simulink model "F550_FaultInjection"  (R2023b)
settings: Solver=FixedStepDiscrete  StartTime=0.0  StopTime=inf  FixedStep=1/100  RelTol=1e-3  EnableMultiTasking=on
undefined symbols (not defined in the file or in its folder): control, IDLEPWM, MC_PITCH_P, MC_PITCHRATE_D, MC_PITCHRATE_I, MC_PITCHRATE_P, MC_ROLL_P, MC_ROLLRATE_D, MC_ROLLRATE_I, MC_ROLLRATE_P, MC_YAW_P, MC_YAWRATE_D, MC_YAWRATE_I, MC_YAWRATE_P, MPC_XY_P, MPC_XY_VEL_MAX, MPC_Z_D, MPC_Z_I, MPC_Z_P, MPC_Z_VEL_D_ACC, MPC_Z_VEL_I_ACC, MPC_Z_VEL_MAX_DN, MPC_Z_VEL_MAX_UP, MPC_Z_VEL_P_ACC, noutputs, output, pitch, pitch_body, roll, roll_body, SampleTime, TargetHardware, thrust_body, timestamp, x, y, yaw, yaw_body, z
libraries: px4lib x45, px4uORBlib x19, slpidlib x10, simulink x9, px4Utilslib x5, simulink_extras x5, px4Sensorslib x3, uavalgslib x3, sharedutil x1, sharedtransform x1
(part 1 of 4)
settings Model: ExtModeTrigDuration=10  Creator=The MathWorks, Inc.  LastModifiedBy=UASG
settings SolverCC: PositivePriorityOrder=on  MaxZcPerStep=1
settings OptimizationCC: StrengthReduction=on  PassReuseOutputArgsAs=Individual arguments  ZeroExternalMemoryAtStartup=off  ZeroInternalMemoryAtStartup=off  MaxStackSize=64  OptimizeBlockOrder=speed  OptimizationPriority=Speed  OptimizationCustomize=off  MultiThreadedLoops=on  EfficientTunableParamExpr=on
settings DebuggingCC: ParameterTunabilityLossMsg=error
settings HardwareCC: ProdBitPerPointer=32  ProdBitPerSizeT=32  ProdBitPerPtrDiffT=32  ProdLargestAtomicInteger=Long  ProdLargestAtomicFloat=Double  ProdWordSize=32  ProdLongLongMode=on  ProdHWDeviceType=ARM Compatible->ARM Cortex
settings ModelReferenceCC: EnableRefExpFcnMdlSchedulingChecks=on
settings SFSimCC: MATLABDynamicMemAlloc=off  SimTargetLang=C++
settings RTWCC: Description=Embedded Coder  SystemTargetFile=ert.tlc  HardwareBoard=PX4 Cube Orange  TLCOptions="-aInlineSetEventsForThisBaseRateFcn=TLC_FALSE -aSuppressMultiTaskScheduler=TLC_FALSE  -aRateBasedStepFcn=0"  TemplateMakefile=ert_default_tmf  GenerateReport=on  Toolchain=GNU Tools for PX4 Autopilots  BuildConfiguration=Faster Runs  LaunchReport=on  TargetLang=C++  DLArmComputeVersion=19.05
settings CodeAppCC: ForceParamTrailComments=on  IgnoreCustomStorageClasses=off  MaxIdLength=63  OperatorAnnotations=on  SimulinkDataObjDesc=on  SFDataObjDesc=on  InsertBlockDesc=on
settings ERTTargetCC: ExtModeTransport=3  ExtModeStaticAlloc=on  ExtModeStaticAllocSize=1024  ExtModeMexFile=ext_xcp  ExtModeIntrfLevel=Level2 - Open

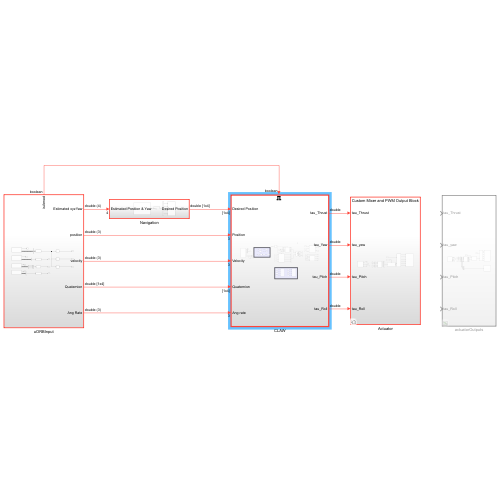
[thumbnail: Simulink's stored preview of the top-level diagram]
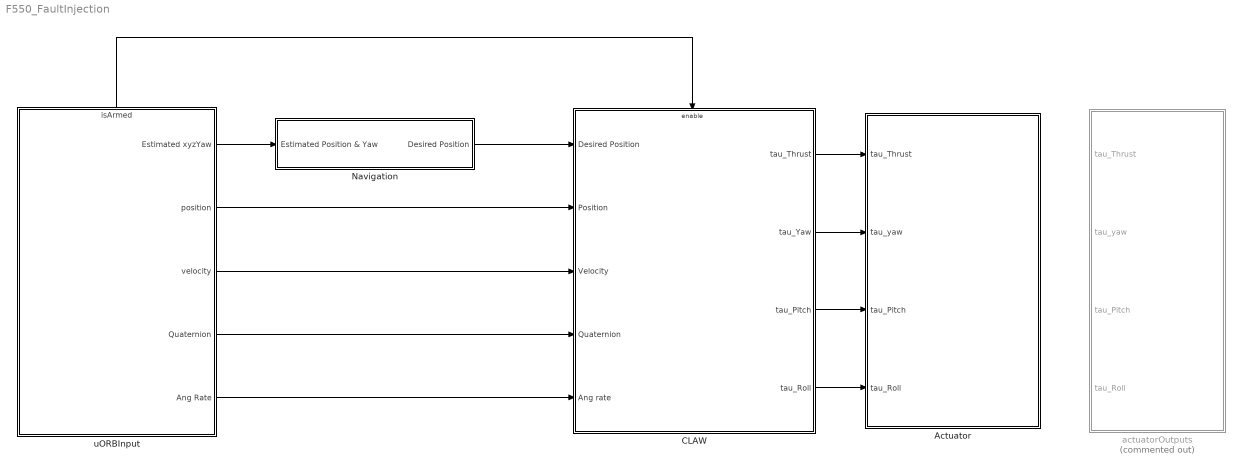
== system F550_FaultInjection ==
  Actuator : Subsystem  Variant=on
  CLAW : Subsystem  RTWFcnName=CLAW
      settings: RTWSystemCode=Nonreusable function  RTWFcnNameOpts=Use subsystem name  RTWFileNameOpts=Use subsystem name
  Navigation : Subsystem
      settings: RTWSystemCode=Nonreusable function  RTWFcnNameOpts=Use subsystem name  RTWFileNameOpts=Use subsystem name
  actuatorOutputs : Subsystem  Commented=on  TreatAsAtomicUnit=on
      settings: RTWSystemCode=Nonreusable function  RTWFcnNameOpts=Use subsystem name  RTWFileNameOpts=Use subsystem name
  uORBInput : Subsystem
      settings: RTWSystemCode=Nonreusable function  RTWFcnNameOpts=Use subsystem name  RTWFileNameOpts=Use subsystem name  PortSchema="{\"entries\":[{\"content\":{\"sides\":[{\"content\":{},\"type\":\"ConnectorPlacement.EquallySpacedRectSide\",\"uuid\":\"c9847de1-a0fb-4f12-b9ba-7a711e150495\"},{\"content\":{\"connectorIds\":[\"Out1\",\"Out2\",\"Out3\",\"Out4\",\"Out5\"],\"side\":\"RIGHT\"},\"type\":\"ConnectorPlacement.EquallySpacedRectSide\",\"uuid\":\"c0766eaa-9e51-4014-aa9e-b3d4f69fc081\"},{\"content\":{\"connectorIds\":[\"Out6\"],\"side\":\"TOP\"},\"type\":\"ConnectorPlacement.EquallySpacedRectSide\",\"uuid\":\"9ded9b51-a7f6-4f6f-b66b-95ea3c1db3ad\"}]},\"type\":\"ConnectorPlacement.EquallySpacedConnector\",\"uuid\":\"83553f6c-d7c4-4220-9d3b-5711d4bd470c\"}],\"packageUris\":[\"http://schema.mathworks.com/mf0/Connector/R2020b\"],\"version\":\"1.0\"}"
  wires:
  uORBInput/1(Estimated xyzYaw) -> Navigation/1(Estimated Position & Yaw)
  CLAW/4(tau_Roll) -> Actuator/4(tau_Roll)
  CLAW/3(tau_Pitch) -> Actuator/3(tau_Pitch)
  CLAW/2(tau_Yaw) -> Actuator/2(tau_yaw)
  CLAW/1(tau_Thrust) -> Actuator/1(tau_Thrust)
  Navigation/1(Desired Position) -> CLAW/1(Desired Position)
  uORBInput/2(position) -> CLAW/2(Position)
  uORBInput/3(velocity) -> CLAW/3(Velocity)
  uORBInput/4(Quaternion) -> CLAW/4(Quaternion)
  uORBInput/5(Ang Rate) -> CLAW/5(Ang rate)
  uORBInput/6(isArmed) -> CLAW/Enable

== system F550_FaultInjection/Actuator ==
  tau_Thrust : Inport
  tau_yaw : Inport  Port=2
  tau_Pitch : Inport  Port=3
  tau_Roll : Inport  Port=4
  Custom Mixer and PWM Output Block : Subsystem  VariantControl=useCustomMixer == true
  PX4 Mixer and actuator_controls_0 topic : Subsystem  VariantControl=useCustomMixer == false

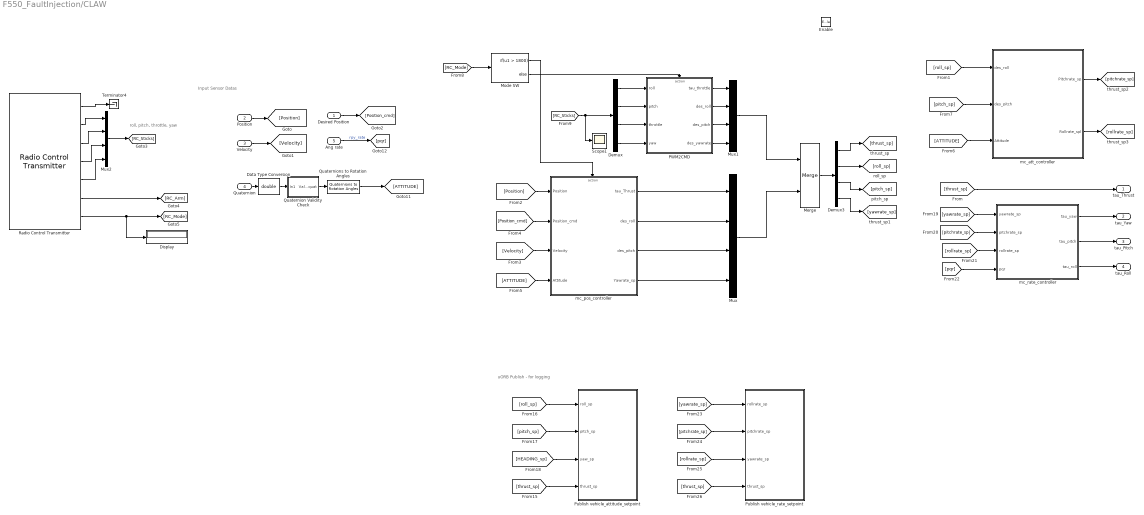
== system F550_FaultInjection/CLAW ==
  note: roll, pitch, throttle, yaw
  note: Input Sensor Datas
  note: uORB Publish - for logging
  Desired Position : Inport
  Position : Inport  Port=2
  Velocity : Inport  Port=3
  Quaternion : Inport  Port=4
  Ang rate : Inport  Port=5
  Enable : EnablePort
  Data Type Conversion : DataTypeConversion  OutDataTypeStr=double  SaturateOnIntegerOverflow=off  RndMeth=Floor
  Demux : Demux
  Demux3 : Demux
  Display : Display
  Merge : Merge
  Mode SW : If  IfExpression=u1 > 1800
  Mux : Mux
  Mux1 : Mux
  Mux2 : Mux
  PWM2CMD : Subsystem
  Publish vehicle_attitude_setpoint : Subsystem
  Publish vehicle_rate_setpoint : Subsystem
  Quaternion Validity Check : Subsystem
  Quaternions to Rotation Angles : sharedtransform/Quaternions to Rotation Angles  rotationOrder=ZYX  aMode=aMode
  Radio Control Transmitter : px4Sensorslib/Radio Control Transmitter  channel1=on  channel2=on  channel3=on  channel4=on  channel5=on  channel6=on  channel7=off  channel8=off  channel_count=off  rssi=off  rc_input_source=off  timestamp_last_signal=off  time_stamp=off  sampleTime=-1  BlockingMode=off  BlockTimeout=5
  Scope1 : Scope
  Terminator4 : Terminator
  mc_att_controller : Subsystem
      settings: RTWSystemCode=Nonreusable function  RTWFcnNameOpts=Use subsystem name  RTWFileNameOpts=Use subsystem name
  mc_pos_controller : Subsystem
      settings: RTWSystemCode=Nonreusable function  RTWFcnNameOpts=Use subsystem name  RTWFileNameOpts=Use subsystem name
  mc_rate_controller : Subsystem
      settings: RTWSystemCode=Nonreusable function  RTWFcnNameOpts=Use subsystem name  RTWFileNameOpts=Use subsystem name
  tau_Thrust : Outport
  tau_Yaw : Outport  Port=2
  tau_Pitch : Outport  Port=3
  tau_Roll : Outport  Port=4
  wires:
  [rollrate_sp] -> Publish vehicle_rate_setpoint/3(yawrate_sp)
  [thrust_sp] -> Publish vehicle_rate_setpoint/4(thrust_sp)
  [yawrate_sp] -> Publish vehicle_rate_setpoint/1(rollrate_sp)
  [yawrate_sp] -> mc_rate_controller/1(yawrate_sp)
  Position/1 -> [Position]
  [pqr] -> mc_rate_controller/4(pqr)
  mc_rate_controller/3(tau_roll) -> tau_Roll/1
  [pitchrate_sp] -> mc_rate_controller/2(pitchrate_sp)
  mc_rate_controller/1(tau_yaw) -> tau_Yaw/1
  mc_att_controller/1(Pitchrate_sp) -> [pitchrate_sp]
  [thrust_sp] -> Publish vehicle_attitude_setpoint/4(thrust_sp)
  [pitchrate_sp] -> Publish vehicle_rate_setpoint/2(pitchrate_sp)
  Quaternion/1 -> Data Type Conversion/1
  mc_rate_controller/2(tau_pitch) -> tau_Pitch/1
  Desired Position/1 -> [Position_cmd]
  Ang rate/1 -> [pqr]  "rpy_rate"
  [thrust_sp] -> tau_Thrust/1
  [rollrate_sp] -> mc_rate_controller/3(rollrate_sp)
  Velocity/1 -> [Velocity]
  mc_att_controller/2(Rollrate_spl) -> [rollrate_sp]
  Quaternion Validity Check/1(Valid quat) -> Quaternions to Rotation Angles/1
  [pitch_sp] -> Publish vehicle_attitude_setpoint/2(pitch_sp)
  [HEADING_sp] -> Publish vehicle_attitude_setpoint/3(yaw_sp)
  [roll_sp] -> Publish vehicle_attitude_setpoint/1(roll_sp)
  Data Type Conversion/1 -> Quaternion Validity Check/1(In1)
  Merge/1 -> Demux3/1
  Demux3/1 -> [thrust_sp]
  Demux3/2 -> [roll_sp]
  Demux3/3 -> [pitch_sp]
  Demux3/4 -> [yawrate_sp]
  [Position] -> mc_pos_controller/1(Position)
  [Velocity] -> mc_pos_controller/3(Velocity)
  [Position_cmd] -> mc_pos_controller/2(Position_cmd)
  [ATTITUDE] -> mc_pos_controller/4(Attitude)
  mc_pos_controller/1(tau_Thrust) -> Mux/1
  mc_pos_controller/2(des_roll) -> Mux/2
  mc_pos_controller/3(des_pitch) -> Mux/3
  mc_pos_controller/4(Yawrate_sp) -> Mux/4
  Mux/1 -> Merge/2
  Mux1/1 -> Merge/1
  [roll_sp] -> mc_att_controller/1(des_roll)
  [ATTITUDE] -> mc_att_controller/3(Attitude)
  [pitch_sp] -> mc_att_controller/2(des_pitch)
  PWM2CMD/1(tau_throttle) -> Mux1/1
  PWM2CMD/2(des_roll) -> Mux1/2
  PWM2CMD/3(des_pitch) -> Mux1/3
  PWM2CMD/4(des_yawrate) -> Mux1/4
  Quaternions to Rotation Angles/1 -> [ATTITUDE]
  [RC_Mode] -> Mode SW/1
  Radio Control Transmitter/6 -> [RC_Arm]
  Radio Control Transmitter/1 -> Terminator4/1
  Radio Control Transmitter/7 -> Display/1, [RC_Mode]
  Radio Control Transmitter/2 -> Mux2/1
  Radio Control Transmitter/3 -> Mux2/2
  Radio Control Transmitter/4 -> Mux2/3
  Radio Control Transmitter/5 -> Mux2/4
  Mux2/1 -> [RC_Sticks]
  Demux/1 -> PWM2CMD/1(roll)
  Demux/2 -> PWM2CMD/2(pitch)
  Demux/3 -> PWM2CMD/3(throttle)
  Demux/4 -> PWM2CMD/4(yaw)
  [RC_Sticks] -> Scope1/1, Demux/1
  Mode SW/2 -> PWM2CMD/Action
  Mode SW/1 -> mc_pos_controller/Action

== system F550_FaultInjection/Navigation ==
  Estimated Position & Yaw : Inport
  Demux : Demux
  Quadcopter Navigation Algorithm : Subsystem  Variant=on
  uORB Publish : Subsystem
  Desired Position : Outport
  wires:
  Quadcopter Navigation Algorithm/1(Desired Position) -> Demux/1, Desired Position/1
  Estimated Position & Yaw/1 -> Quadcopter Navigation Algorithm/1(Current Position)
  Demux/1 -> uORB Publish/1(x_sp)
  Demux/2 -> uORB Publish/2(y_sp)
  Demux/3 -> uORB Publish/3(z_sp)
  Demux/4 -> uORB Publish/4(heading_sp)

== system F550_FaultInjection/actuatorOutputs ==
  tau_Thrust : Inport
  tau_yaw : Inport  Port=2
  tau_Pitch : Inport  Port=3
  tau_Roll : Inport  Port=4
  Emergency Kill : Subsystem
  Fault Injection Module : Subsystem  Variant=on
  Gain : Gain  Gain=5
  Gain1 : Gain  Gain=5
  Gain2 : Gain  Gain=10
  MATLAB Function : MATLAB Function  TreatAsAtomicUnit=on
  Mux : Mux  Inputs=6
  Mux1 : Mux
  Radio Control Transmitter : px4Sensorslib/Radio Control Transmitter  channel1=off  channel2=off  channel3=off  channel4=off  channel5=off  channel6=on  channel7=on  channel8=off  channel_count=off  rssi=off  rc_input_source=off  timestamp_last_signal=off  time_stamp=off  sampleTime=-1  BlockingMode=off  BlockTimeout=5
  Saturation : Saturate  UpperLimit=1  LowerLimit=0
  Saturation1 : Saturate  UpperLimit=1  LowerLimit=-1
  Saturation2 : Saturate  UpperLimit=1  LowerLimit=-1
  Saturation3 : Saturate  UpperLimit=1  LowerLimit=-1
  Terminator : Terminator
  uORB_actuator_controls : Subsystem
  uORB_actuator_outputs : Subsystem
  wires:
  MATLAB Function/1(M1) -> Mux/1
  Radio Control Transmitter/1 -> Terminator/1
  MATLAB Function/2(M2) -> Mux/2
  tau_Thrust/1 -> Saturation/1  "thrust cmd"
  tau_Pitch/1 -> Gain1/1  "pitch cmd"
  MATLAB Function/3(M3) -> Mux/3
  [Kill] -> Emergency Kill/1(Kill)
  MATLAB Function/6(M6) -> Mux/6
  tau_yaw/1 -> Gain2/1
  Radio Control Transmitter/2 -> [InjectFault]
  Radio Control Transmitter/3 -> [Kill]
  tau_Roll/1 -> Gain/1  "roll_cmd"
  MATLAB Function/4(M4) -> Mux/4
  MATLAB Function/5(M5) -> Mux/5
  [InjectFault] -> Fault Injection Module/1(Inject Fault)
  Mux/1 -> Fault Injection Module/2(PWM_IN)
  Fault Injection Module/1(PWM_OUT) -> Emergency Kill/2(PWM_IN)
  Mux1/1 -> uORB_actuator_controls/1(actuator_control_out)
  Saturation/1 -> Mux1/4, MATLAB Function/4(Thrust)
  Saturation1/1 -> Mux1/3, MATLAB Function/3(Yaw)
  Saturation2/1 -> Mux1/2, MATLAB Function/2(Pitch)
  Saturation3/1 -> Mux1/1, MATLAB Function/1(Roll)
  Gain/1 -> Saturation3/1
  Gain1/1 -> Saturation2/1
  Gain2/1 -> Saturation1/1
  Emergency Kill/1(M1_OUT) -> uORB_actuator_outputs/1(Ch1)
  Emergency Kill/2(M2_OUT) -> uORB_actuator_outputs/2(Ch2)
  Emergency Kill/3(M3_OUT) -> uORB_actuator_outputs/3(Ch3)
  Emergency Kill/4(M4_OUT) -> uORB_actuator_outputs/4(Ch4)
  Emergency Kill/5(M5_OUT) -> uORB_actuator_outputs/5(Ch5)
  Emergency Kill/6(M6_OUT) -> uORB_actuator_outputs/6(Ch6)

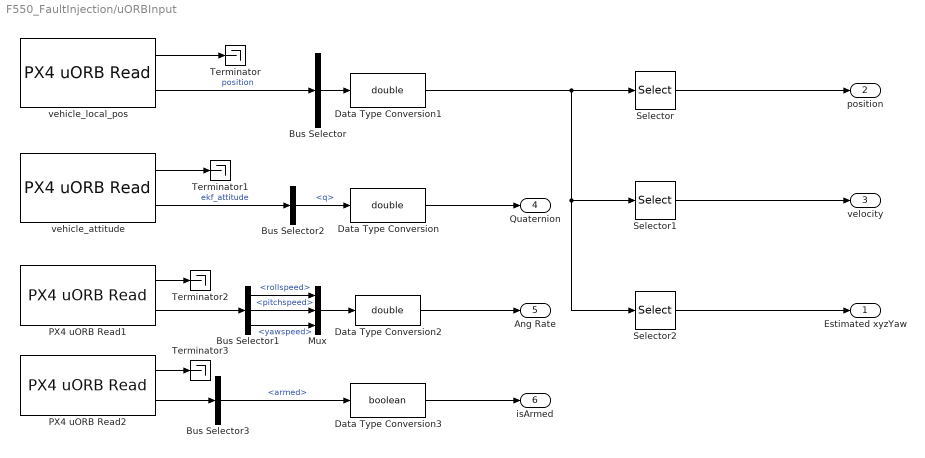
== system F550_FaultInjection/uORBInput ==
  Bus Selector : BusSelector  OutputSignals=x,y,z,vx,vy,vz,heading  OutputAsBus=on
  Bus Selector1 : BusSelector  OutputSignals=rollspeed,pitchspeed,yawspeed
  Bus Selector2 : BusSelector  OutputSignals=q
  Bus Selector3 : BusSelector  OutputSignals=armed
  Data Type Conversion : DataTypeConversion  OutDataTypeStr=double  SaturateOnIntegerOverflow=off  RndMeth=Floor
  Data Type Conversion1 : DataTypeConversion  OutDataTypeStr=double  SaturateOnIntegerOverflow=off  RndMeth=Floor
  Data Type Conversion2 : DataTypeConversion  OutDataTypeStr=double  SaturateOnIntegerOverflow=off  RndMeth=Floor
  Data Type Conversion3 : DataTypeConversion  OutDataTypeStr=boolean  SaturateOnIntegerOverflow=off  RndMeth=Floor
  Mux : Mux  Inputs=3
  PX4 uORB Read1 : px4uORBlib/PX4 uORB Read  uORBTopic=vehicle_odometry  selectInstance=vehicle_odometry  SampleTime=-1  BlockingMode=off  BlockTimeout=1e-3
  PX4 uORB Read2 : px4uORBlib/PX4 uORB Read  uORBTopic=actuator_armed  selectInstance=actuator_armed  SampleTime=-1  BlockingMode=off  BlockTimeout=1e-3
  Selector : Selector  InputPortWidth=7  IndexOptions=Index vector (dialog)  Indices=[1:3]  OutputSizes=1
  Selector1 : Selector  InputPortWidth=7  IndexOptions=Index vector (dialog)  Indices=[4:6]  OutputSizes=1
  Selector2 : Selector  InputPortWidth=7  IndexOptions=Index vector (dialog)  Indices=[1 2 3 7]  OutputSizes=1
  Terminator{,1..3} (4 alike) : Terminator
  vehicle_attitude : px4uORBlib/PX4 uORB Read  uORBTopic=vehicle_attitude  selectInstance=vehicle_attitude  SampleTime=-1  BlockingMode=off  BlockTimeout=1e-3
  vehicle_local_pos : px4uORBlib/PX4 uORB Read  uORBTopic=vehicle_local_position  selectInstance=vehicle_local_position  SampleTime=-1  BlockingMode=off  BlockTimeout=1e-3
  Estimated xyzYaw : Outport
  position : Outport  Port=2
  velocity : Outport  Port=3
  Quaternion : Outport  Port=4
  Ang Rate : Outport  Port=5
  isArmed : Outport  Port=6
  wires:
  Bus Selector2/1 -> Data Type Conversion/1  "<q>"
  vehicle_local_pos/2 -> Bus Selector/1  "position"
  Data Type Conversion1/1 -> Selector1/1, Selector2/1, Selector/1
  vehicle_attitude/1 -> Terminator1/1
  vehicle_attitude/2 -> Bus Selector2/1  "ekf_attitude"
  vehicle_local_pos/1 -> Terminator/1
  Bus Selector/1 -> Data Type Conversion1/1
  PX4 uORB Read1/1 -> Terminator2/1
  PX4 uORB Read1/2 -> Bus Selector1/1
  Mux/1 -> Data Type Conversion2/1
  PX4 uORB Read2/1 -> Terminator3/1
  Bus Selector3/1 -> Data Type Conversion3/1  "<armed>"
  PX4 uORB Read2/2 -> Bus Selector3/1
  Bus Selector1/1 -> Mux/1  "<rollspeed>"
  Bus Selector1/2 -> Mux/2  "<pitchspeed>"
  Bus Selector1/3 -> Mux/3  "<yawspeed>"
  Selector/1 -> position/1
  Selector1/1 -> velocity/1
  Selector2/1 -> Estimated xyzYaw/1
  Data Type Conversion/1 -> Quaternion/1
  Data Type Conversion2/1 -> Ang Rate/1
  Data Type Conversion3/1 -> isArmed/1

== system F550_FaultInjection/Actuator/Custom Mixer and PWM Output Block ==
  tau_Thrust : Inport
  tau_yaw : Inport  Port=2
  tau_Pitch : Inport  Port=3
  tau_Roll : Inport  Port=4
  Emergency Kill : Subsystem
  Fault_Injection : Subsystem
      settings: PortSchema="{\"entries\":[{\"content\":{\"sides\":[{\"content\":{\"connectorIds\":[\"In1\"]},\"type\":\"ConnectorPlacement.EquallySpacedRectSide\",\"uuid\":\"fab26c65-8d77-46b7-b375-2033d08e8306\"},{\"content\":{\"connectorIds\":[\"Out1\"],\"side\":\"RIGHT\"},\"type\":\"ConnectorPlacement.EquallySpacedRectSide\",\"uuid\":\"bc3f50bd-e170-4b75-8089-4f92da68e83e\"},{\"content\":{\"connectorIds\":[\"In2\"],\"side\":\"TOP\"},\"type\":\"ConnectorPlacement.EquallySpacedRectSide\",\"uuid\":\"873ada90-6f93-48ab-a701-a52d28357753\"}]},\"type\":\"ConnectorPlacement.EquallySpacedConnector\",\"uuid\":\"201be8b3-bff4-4924-8e0c-28e5fee33d1c\"}],\"packageUris\":[\"http://schema.mathworks.com/mf0/Connector/R2020b\"],\"version\":\"1.0\"}"
  Gain : Gain  Gain=5
  Gain1 : Gain  Gain=5
  Gain2 : Gain  Gain=10
  Gain3 : Gain
  MATLAB Function : MATLAB Function  TreatAsAtomicUnit=on
  Mux : Mux  Inputs=6
  Radio Control Transmitter : px4Sensorslib/Radio Control Transmitter  channel1=off  channel2=off  channel3=off  channel4=off  channel5=off  channel6=off  channel7=on  channel8=on  channel_count=off  rssi=off  rc_input_source=off  timestamp_last_signal=off  time_stamp=off  sampleTime=-1  BlockingMode=off  BlockTimeout=5
  Subsystem : Subsystem
  Terminator : Terminator
  wires:
  Radio Control Transmitter/2 -> [Kill]
  [InjectFault] -> Fault_Injection/2(Inject Fault)
  Fault_Injection/1(PWM_OUT) -> Emergency Kill/2(PWM_IN)
  [Kill] -> Emergency Kill/1(Kill)
  Radio Control Transmitter/3 -> [InjectFault]
  Radio Control Transmitter/1 -> Terminator/1
  Emergency Kill/2(M2_OUT) -> Subsystem/2(Ch2)
  Emergency Kill/3(M3_OUT) -> Subsystem/3(Ch3)
  Emergency Kill/4(M4_OUT) -> Subsystem/4(Ch4)
  Emergency Kill/5(M5_OUT) -> Subsystem/5(Ch5)
  Emergency Kill/6(M6_OUT) -> Subsystem/6(Ch6)
  Emergency Kill/1(M1_OUT) -> Subsystem/1(Ch1)
  tau_Thrust/1 -> Gain3/1  "thrust cmd"
  tau_Roll/1 -> Gain/1  "roll_cmd"
  tau_Pitch/1 -> Gain1/1  "pitch cmd"
  tau_yaw/1 -> Gain2/1
  MATLAB Function/1(M1) -> Mux/1
  MATLAB Function/2(M2) -> Mux/2
  MATLAB Function/3(M3) -> Mux/3
  MATLAB Function/4(M4) -> Mux/4
  MATLAB Function/5(M5) -> Mux/5
  MATLAB Function/6(M6) -> Mux/6
  Mux/1 -> Fault_Injection/1(PWM_IN)
  Gain/1 -> MATLAB Function/1(Roll)
  Gain1/1 -> MATLAB Function/2(Pitch)
  Gain2/1 -> MATLAB Function/3(Yaw)
  Gain3/1 -> MATLAB Function/4(Thrust)

== system F550_FaultInjection/Actuator/PX4 Mixer and actuator_controls_0 topic ==
  tau_Thrust : Inport
  tau_yaw : Inport  Port=2
  tau_Pitch : Inport  Port=3
  tau_Roll : Inport  Port=4
  Armed : Inport  Port=5
  Bus Assignment : BusAssignment  AssignedSignals=control
  Constant : Constant  Value=zeros(4,1)
  Data Type Conversion : DataTypeConversion  SaturateOnIntegerOverflow=off  RndMeth=Floor
  Mux : Mux  Inputs=5
  PX4 uORB Message : px4uORBlib/PX4 uORB Message  uORBTopic=actuator_controls  SampleTime=inf  selectInstance=vehicle_gps_position
  PX4 uORB Write : px4uORBlib/PX4 uORB Write  uORBTopic=actuator_controls  selectInstance=actuator_controls_0  MessageQueueLen=1
  Terminator : Terminator
  wires:
  Bus Assignment/1 -> PX4 uORB Write/1
  tau_yaw/1 -> Mux/3
  Data Type Conversion/1 -> Bus Assignment/2
  tau_Roll/1 -> Mux/1  "roll_cmd"
  PX4 uORB Message/1 -> Bus Assignment/1
  Mux/1 -> Data Type Conversion/1
  Constant/1 -> Mux/5
  tau_Pitch/1 -> Mux/2  "pitch cmd"
  tau_Thrust/1 -> Mux/4  "thrust cmd"
  Armed/1 -> Terminator/1

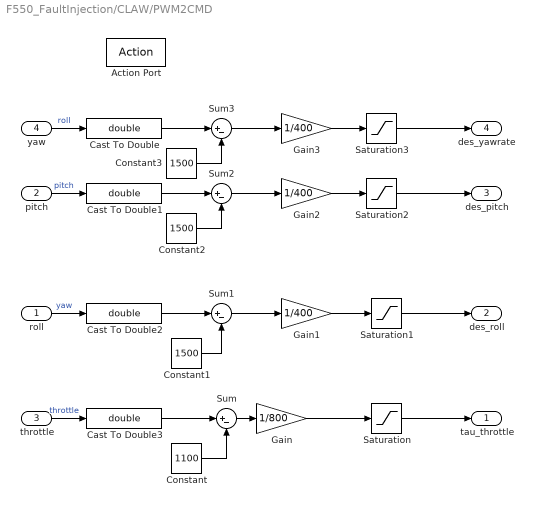
== system F550_FaultInjection/CLAW/PWM2CMD ==
  roll : Inport
  pitch : Inport  Port=2
  throttle : Inport  Port=3
  yaw : Inport  Port=4
  Action Port : ActionPort  ActionPortLabel=else
  Cast To Double{,1..3} (4 alike) : DataTypeConversion  OutDataTypeStr=double  SaturateOnIntegerOverflow=off  RndMeth=Floor
  Constant : Constant  Value=1100
  Constant1 : Constant  Value=1500
  Constant2 : Constant  Value=1500
  Constant3 : Constant  Value=1500
  Gain : Gain  Gain=1/800
  Gain1 : Gain  Gain=1/400
  Gain2 : Gain  Gain=1/400
  Gain3 : Gain  Gain=1/400
  Saturation : Saturate  UpperLimit=1  LowerLimit=0
  Saturation1 : Saturate  UpperLimit=1  LowerLimit=-1
  Saturation2 : Saturate  UpperLimit=1  LowerLimit=-1
  Saturation3 : Saturate  UpperLimit=1  LowerLimit=-1
  Sum{,1..3} (4 alike) : Sum  Inputs=|+-
  tau_throttle : Outport
  des_roll : Outport  Port=2
  des_pitch : Outport  Port=3
  des_yawrate : Outport  Port=4
  wires:
  Gain/1 -> Saturation/1
  Constant1/1 -> Sum1/2
  throttle/1 -> Cast To Double3/1  "throttle"
  yaw/1 -> Cast To Double/1  "roll"
  Constant3/1 -> Sum3/2
  Gain2/1 -> Saturation2/1
  pitch/1 -> Cast To Double1/1  "pitch"
  Constant2/1 -> Sum2/2
  roll/1 -> Cast To Double2/1  "yaw"
  Sum1/1 -> Gain1/1
  Sum2/1 -> Gain2/1
  Gain3/1 -> Saturation3/1
  Constant/1 -> Sum/2
  Sum/1 -> Gain/1
  Sum3/1 -> Gain3/1
  Gain1/1 -> Saturation1/1
  Saturation3/1 -> des_yawrate/1
  Saturation2/1 -> des_pitch/1
  Saturation1/1 -> des_roll/1
  Saturation/1 -> tau_throttle/1
  Cast To Double/1 -> Sum3/1
  Cast To Double1/1 -> Sum2/1
  Cast To Double2/1 -> Sum1/1
  Cast To Double3/1 -> Sum/1

== system F550_FaultInjection/CLAW/Publish vehicle_attitude_setpoint ==
  note: bX : Body frame ,X axis
  roll_sp : Inport
  pitch_sp : Inport  Port=2
  yaw_sp : Inport  Port=3
  thrust_sp : Inport  Port=4
  Bus Assignment : BusAssignment  AssignedSignals=timestamp,roll_body,pitch_body,yaw_body,thrust_body
  Data Type Conversion{,1..3} (4 alike) : DataTypeConversion  OutDataTypeStr=single  SaturateOnIntegerOverflow=off  RndMeth=Floor
  Mux : Mux  Inputs=3
  PX4 Timestamp : px4Utilslib/PX4 Timestamp  SampleTime=-1
  PX4 uORB Message : px4uORBlib/PX4 uORB Message  uORBTopic=vehicle_attitude_setpoint  SampleTime=-1  selectInstance=actuator_controls
  PX4 uORB Write : px4uORBlib/PX4 uORB Write  uORBTopic=vehicle_attitude_setpoint  selectInstance=vehicle_attitude_setpoint  MessageQueueLen=1
  thrust_sp_bX : Constant  Value=0
  thrust_sp_bY : Constant  Value=0
  wires:
  PX4 Timestamp/1 -> Bus Assignment/2
  Bus Assignment/1 -> PX4 uORB Write/1
  PX4 uORB Message/1 -> Bus Assignment/1
  roll_sp/1 -> Data Type Conversion/1
  pitch_sp/1 -> Data Type Conversion1/1
  yaw_sp/1 -> Data Type Conversion2/1
  Data Type Conversion/1 -> Bus Assignment/3
  Data Type Conversion1/1 -> Bus Assignment/4
  Data Type Conversion2/1 -> Bus Assignment/5
  thrust_sp_bX/1 -> Mux/1
  thrust_sp_bY/1 -> Mux/2
  thrust_sp/1 -> Mux/3
  Mux/1 -> Data Type Conversion3/1
  Data Type Conversion3/1 -> Bus Assignment/6

== system F550_FaultInjection/CLAW/Publish vehicle_rate_setpoint ==
  note: bX : Body frame ,X axis
  rollrate_sp : Inport
  pitchrate_sp : Inport  Port=2
  yawrate_sp : Inport  Port=3
  thrust_sp : Inport  Port=4
  Bus Assignment : BusAssignment  AssignedSignals=timestamp,roll,pitch,yaw,thrust_body
  Data Type Conversion{,1..3} (4 alike) : DataTypeConversion  OutDataTypeStr=single  SaturateOnIntegerOverflow=off  RndMeth=Floor
  Mux : Mux  Inputs=3
  PX4 Timestamp : px4Utilslib/PX4 Timestamp  SampleTime=-1
  PX4 uORB Message : px4uORBlib/PX4 uORB Message  uORBTopic=vehicle_rates_setpoint  SampleTime=-1  selectInstance=vehicle_rates_setpoint
  PX4 uORB Write : px4uORBlib/PX4 uORB Write  uORBTopic=vehicle_rates_setpoint  selectInstance=vehicle_rates_setpoint  MessageQueueLen=1
  thrust_sp_bX : Constant  Value=0
  thrust_sp_bY : Constant  Value=0
  wires:
  PX4 Timestamp/1 -> Bus Assignment/2
  Bus Assignment/1 -> PX4 uORB Write/1
  PX4 uORB Message/1 -> Bus Assignment/1
  rollrate_sp/1 -> Data Type Conversion/1
  pitchrate_sp/1 -> Data Type Conversion1/1
  yawrate_sp/1 -> Data Type Conversion2/1
  Data Type Conversion/1 -> Bus Assignment/3
  Data Type Conversion1/1 -> Bus Assignment/4
  Data Type Conversion2/1 -> Bus Assignment/5
  thrust_sp_bX/1 -> Mux/1
  thrust_sp_bY/1 -> Mux/2
  thrust_sp/1 -> Mux/3
  Mux/1 -> Data Type Conversion3/1
  Data Type Conversion3/1 -> Bus Assignment/6

== system F550_FaultInjection/CLAW/Quaternion Validity Check ==
  In1 : Inport
  Constant : Constant  Value=[1 0 0 0]  SampleTime=-1
  Quaternion Norm : sharedutil/Quaternion Norm  aMode=aMode
  Switch : Switch  Criteria=u2 > Threshold  SaturateOnIntegerOverflow=off  InputSameDT=off
  Valid quat : Outport
  wires:
  In1/1 -> Quaternion Norm/1, Switch/1
  Quaternion Norm/1 -> Switch/2
  Switch/1 -> Valid quat/1
  Constant/1 -> Switch/3

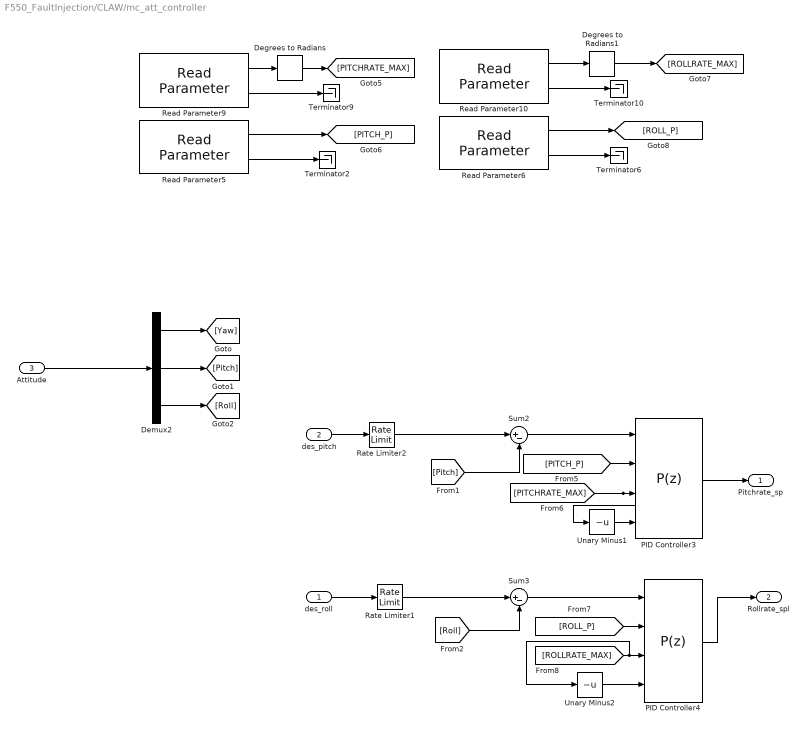
== system F550_FaultInjection/CLAW/mc_att_controller ==
  des_roll : Inport
  des_pitch : Inport  Port=2
  Attitude : Inport  Port=3
  Degrees to Radians : simulink_extras/Transformations/Degrees to Radians
  Degrees to Radians1 : simulink_extras/Transformations/Degrees to Radians
  Demux2 : Demux  Outputs=3
  PID Controller3 : slpidlib/PID Controller  Controller=P  Form=Parallel  TimeDomain=Discrete-time  UseExternalTs=off  SampleTime=-1  IntegratorMethod=Forward Euler  FilterMethod=Forward Euler  ControllerParametersSource=external  P=MC_PITCH_P  I=1  UseKiTs=off  D=0  N=100  UseFilter=on  TunerSelectOption=Transfer Function Based (PID Tuner App)  InitialConditionSource=internal  InitialConditionForIntegrator=0  InitialConditionForFilter=0  DifferentiatorICPrevScaledInput=0  ExternalReset=none  TrackingMode=off  Kt=1  LimitOutput=on  SatLimitsSource=external  UpperSaturationLimit=inf  LowerSaturationLimit=-inf  LinearizeAsGain=on  AntiWindupMode=none  Kb=1  LimitIntegrator=off  UpperIntegratorSaturationLimit=inf  LowerIntegratorSaturationLimit=-inf  POutMin=[]  POutMax=[]  IOutMin=[]  IOutMax=[]  DOutMin=[]  DOutMax=[]  NOutMin=[]  NOutMax=[]  SumOutMin=[]  SumOutMax=[]  SaturationOutMin=[]  SaturationOutMax=[]  PParamMin=[]  PParamMax=[]  IParamMin=[]  IParamMax=[]  DParamMin=[]  DParamMax=[]  NParamMin=[]  NParamMax=[]  KbParamMin=[]  KbParamMax=[]  KtParamMin=[]  KtParamMax=[]  KbOutMin=[]  KbOutMax=[]  KtOutMin=[]  KtOutMax=[]  IntegratorOutMin=[]  IntegratorOutMax=[]  FilterOutMin=[]  FilterOutMax=[]  SumI1OutMin=[]  SumI1OutMax=[]  SumI2OutMin=[]  SumI2OutMax=[]  SumI3OutMin=[]  SumI3OutMax=[]  SumI4OutMin=[]  SumI4OutMax=[]  SumDOutMin=[]  SumDOutMax=[]  DifferentiatorOutMin=[]  DifferentiatorOutMax=[]  FilterDiffOutCoefMin=[]  FilterDiffOutCoefMax=[]  ReciprocalOutMin=[]  ReciprocalOutMax=[]  SumDenOutMin=[]  SumDenOutMax=[]  SumNumOutMin=[]  SumNumOutMax=[]  DivideOutMin=[]  DivideOutMax=[]  UdiffTsProdOutMin=[]  UdiffTsProdOutMax=[]  NTsProdOutMin=[]  NTsProdOutMax=[]  UintegralTsProdOutMin=[]  UintegralTsProdOutMax=[]  UngainTsProdOutMin=[]  UngainTsProdOutMax=[]  ClampingZeroOutDataTypeStr=Inherit: Inherit via back propagation  ClampingZeroOutMin=[]  ClampingZeroOutMax=[]  FilterDenConstantOutDataTypeStr=Inherit: Inherit via back propagation  FilterDenConstantOutMin=[]  FilterDenConstantOutMax=[]  PCopyOutDataTypeStr=Inherit: Inherit via back propagation  PCopyOutMin=[]  PCopyOutMax=[]  NCopyOutDataTypeStr=Inherit: Inherit via back propagation  NCopyOutMin=[]  NCopyOutMax=[]  IntegratorContinuousStateAttributes=''  IntegratorStateMustResolveToSignalObject=off  IntegratorRTWStateStorageClass=Auto  FilterContinuousStateAttributes=''  FilterStateMustResolveToSignalObject=off  FilterRTWStateStorageClass=Auto  ParallelPVariant=ExternalParameters  IdealPVariant=Disabled  IVariant=Disabled  DVariant=Disabled  IntegratorVariant=Disabled  SatVariant=External  AWVariant=Disabled  PCopyVariant=Disabled  TRVariant=Disabled  FdbkBlocksVariant=Forward  IdealPFdbkVariant=Disabled  SatFdbkVariant=Disabled  DerivativeFilterVariant=Disabled  NVariant=Disabled  NCopyVariant=Disabled_SignalSpec  FilterICVariant=Disabled  IntegratorICVariant=Disabled  ExternalResetVariant=Disabled  TRSumVariant=Passthrough  SumFdbkVariant=Disabled  SumVariant=Passthrough_P  TsampFilterVariant=InternalTs  TsampNgainVariant=Passthrough  TsampIntegralVariant=Disabled_SignalSpec  ExternalSaturationOutDataTypeStr=Inherit: Same as second input
  PID Controller4 : slpidlib/PID Controller  Controller=P  Form=Parallel  TimeDomain=Discrete-time  UseExternalTs=off  SampleTime=-1  IntegratorMethod=Forward Euler  FilterMethod=Forward Euler  ControllerParametersSource=external  P=MC_ROLL_P  I=1  UseKiTs=off  D=0  N=100  UseFilter=on  TunerSelectOption=Transfer Function Based (PID Tuner App)  InitialConditionSource=internal  InitialConditionForIntegrator=0  InitialConditionForFilter=0  DifferentiatorICPrevScaledInput=0  ExternalReset=none  TrackingMode=off  Kt=1  LimitOutput=on  SatLimitsSource=external  UpperSaturationLimit=inf  LowerSaturationLimit=-inf  LinearizeAsGain=on  AntiWindupMode=none  Kb=1  LimitIntegrator=off  UpperIntegratorSaturationLimit=inf  LowerIntegratorSaturationLimit=-inf  POutMin=[]  POutMax=[]  IOutMin=[]  IOutMax=[]  DOutMin=[]  DOutMax=[]  NOutMin=[]  NOutMax=[]  SumOutMin=[]  SumOutMax=[]  SaturationOutMin=[]  SaturationOutMax=[]  PParamMin=[]  PParamMax=[]  IParamMin=[]  IParamMax=[]  DParamMin=[]  DParamMax=[]  NParamMin=[]  NParamMax=[]  KbParamMin=[]  KbParamMax=[]  KtParamMin=[]  KtParamMax=[]  KbOutMin=[]  KbOutMax=[]  KtOutMin=[]  KtOutMax=[]  IntegratorOutMin=[]  IntegratorOutMax=[]  FilterOutMin=[]  FilterOutMax=[]  SumI1OutMin=[]  SumI1OutMax=[]  SumI2OutMin=[]  SumI2OutMax=[]  SumI3OutMin=[]  SumI3OutMax=[]  SumI4OutMin=[]  SumI4OutMax=[]  SumDOutMin=[]  SumDOutMax=[]  DifferentiatorOutMin=[]  DifferentiatorOutMax=[]  FilterDiffOutCoefMin=[]  FilterDiffOutCoefMax=[]  ReciprocalOutMin=[]  ReciprocalOutMax=[]  SumDenOutMin=[]  SumDenOutMax=[]  SumNumOutMin=[]  SumNumOutMax=[]  DivideOutMin=[]  DivideOutMax=[]  UdiffTsProdOutMin=[]  UdiffTsProdOutMax=[]  NTsProdOutMin=[]  NTsProdOutMax=[]  UintegralTsProdOutMin=[]  UintegralTsProdOutMax=[]  UngainTsProdOutMin=[]  UngainTsProdOutMax=[]  ClampingZeroOutDataTypeStr=Inherit: Inherit via back propagation  ClampingZeroOutMin=[]  ClampingZeroOutMax=[]  FilterDenConstantOutDataTypeStr=Inherit: Inherit via back propagation  FilterDenConstantOutMin=[]  FilterDenConstantOutMax=[]  PCopyOutDataTypeStr=Inherit: Inherit via back propagation  PCopyOutMin=[]  PCopyOutMax=[]  NCopyOutDataTypeStr=Inherit: Inherit via back propagation  NCopyOutMin=[]  NCopyOutMax=[]  IntegratorContinuousStateAttributes=''  IntegratorStateMustResolveToSignalObject=off  IntegratorRTWStateStorageClass=Auto  FilterContinuousStateAttributes=''  FilterStateMustResolveToSignalObject=off  FilterRTWStateStorageClass=Auto  ParallelPVariant=ExternalParameters  IdealPVariant=Disabled  IVariant=Disabled  DVariant=Disabled  IntegratorVariant=Disabled  SatVariant=External  AWVariant=Disabled  PCopyVariant=Disabled  TRVariant=Disabled  FdbkBlocksVariant=Forward  IdealPFdbkVariant=Disabled  SatFdbkVariant=Disabled  DerivativeFilterVariant=Disabled  NVariant=Disabled  NCopyVariant=Disabled_SignalSpec  FilterICVariant=Disabled  IntegratorICVariant=Disabled  ExternalResetVariant=Disabled  TRSumVariant=Passthrough  SumFdbkVariant=Disabled  SumVariant=Passthrough_P  TsampFilterVariant=InternalTs  TsampNgainVariant=Passthrough  TsampIntegralVariant=Disabled_SignalSpec  ExternalSaturationOutDataTypeStr=Inherit: Same as second input
  Rate Limiter1 : RateLimiter  RisingSlewLimit=180*pi/180  FallingSlewLimit=-180*pi/180  SampleTimeMode=inherited
  Rate Limiter2 : RateLimiter  RisingSlewLimit=180*pi/180  FallingSlewLimit=-180*pi/180  SampleTimeMode=inherited
  Read Parameter10 : px4lib/Read Parameter  ParameterName=SL_ROLLRATE_MAX  DataType=FLOAT  SampleTime=-1
  Read Parameter5 : px4lib/Read Parameter  ParameterName=SL_PITCH_P  DataType=FLOAT  SampleTime=-1
  Read Parameter6 : px4lib/Read Parameter  ParameterName=SL_ROLL_P  DataType=FLOAT  SampleTime=-1
  Read Parameter9 : px4lib/Read Parameter  ParameterName=SL_PITCHRATE_MAX  DataType=FLOAT  SampleTime=-1
  Sum2 : Sum  Inputs=|+-
  Sum3 : Sum  Inputs=|+-
  Terminator{2,6,9..10} (4 alike) : Terminator
  Unary Minus1 : UnaryMinus
  Unary Minus2 : UnaryMinus
  Pitchrate_sp : Outport
  Rollrate_spl : Outport  Port=2
  wires:
  Sum2/1 -> PID Controller3/1
  Sum3/1 -> PID Controller4/1
  Attitude/1 -> Demux2/1
  des_roll/1 -> Rate Limiter1/1
  Rate Limiter1/1 -> Sum3/1
  Rate Limiter2/1 -> Sum2/1
  des_pitch/1 -> Rate Limiter2/1
  PID Controller3/1 -> Pitchrate_sp/1
  PID Controller4/1 -> Rollrate_spl/1
  Demux2/1 -> [Yaw]
  Demux2/2 -> [Pitch]
  Demux2/3 -> [Roll]
  [Pitch] -> Sum2/2
  [Roll] -> Sum3/2
  Read Parameter6/1 -> [ROLL_P]
  Read Parameter5/1 -> [PITCH_P]
  Read Parameter10/2 -> Terminator10/1
  Read Parameter9/2 -> Terminator9/1
  Read Parameter10/1 -> Degrees to Radians1/1
  Read Parameter9/1 -> Degrees to Radians/1
  Read Parameter5/2 -> Terminator2/1
  Read Parameter6/2 -> Terminator6/1
  [PITCH_P] -> PID Controller3/2
  [PITCHRATE_MAX] -> Unary Minus1/1, PID Controller3/3
  Unary Minus1/1 -> PID Controller3/4
  [ROLL_P] -> PID Controller4/2
  [ROLLRATE_MAX] -> Unary Minus2/1, PID Controller4/3
  Unary Minus2/1 -> PID Controller4/4
  Degrees to Radians1/1 -> [ROLLRATE_MAX]
  Degrees to Radians/1 -> [PITCHRATE_MAX]
